simulink subsystem "induction_motor_model"  (R2024b)
settings: Solver=VariableStepAuto  StartTime=0.0  StopTime=10.0  RelTol=1e-3
model mask{A=400, f=50}
  mask prompts: A "Amplitude (V)"; f "Frequency (Hz)"
settings Model: Creator=antoinedaniel  LastModifiedBy=antoinedaniel

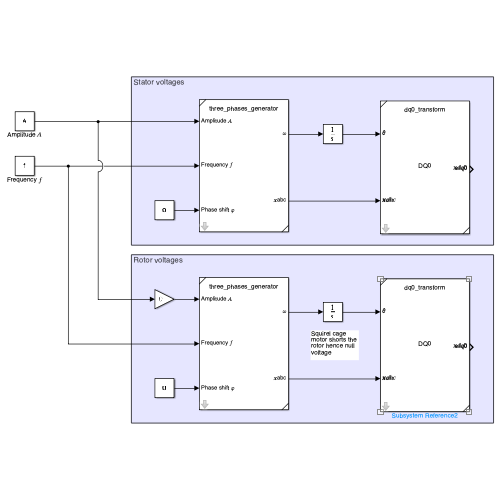
[thumbnail: Simulink's stored preview of the top-level diagram]
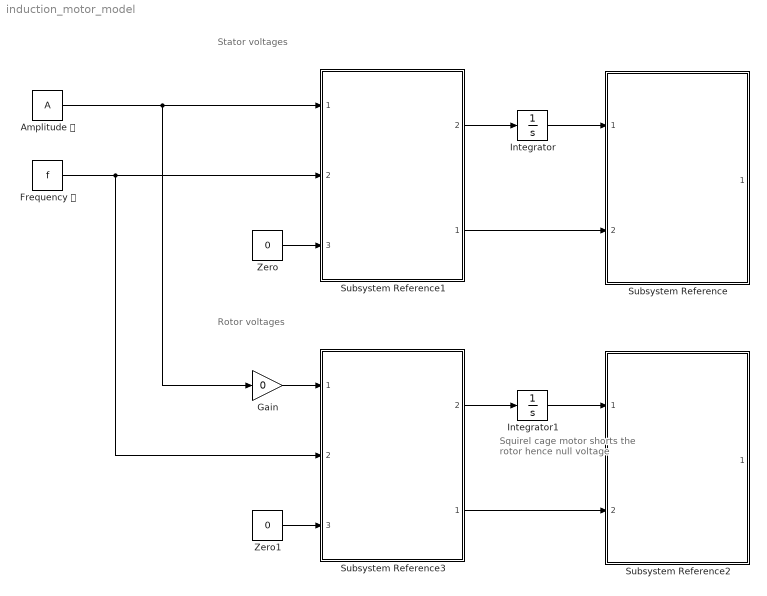
== system induction_motor_model ==
  note: Stator voltages
  note: Squirel cage motor shorts the rotor hence null voltage
  note: Rotor voltages
  Amplitude 𝐴 : Constant  Value=A
  Frequency 𝑓 : Constant  Value=f
  Gain : Gain  Gain=0
  Integrator : Integrator
  Integrator1 : Integrator
  Subsystem Reference : Subsystem  ReferencedSubsystem=dq0_transform  SignConv=Negative
  Subsystem Reference1 : Subsystem  ReferencedSubsystem=three_phases_generator
      settings: PortSchema="{\"entries\":[{\"content\":{\"sides\":[{\"content\":{\"connectorIds\":[\"In1\",\"In2\",\"In3\"]},\"type\":\"ConnectorPlacement.EquallySpacedRectSide\",\"uuid\":\"83e992db-efbf-4d18-ab7d-fa4d5e1c88d1\"},{\"content\":{\"connectorIds\":[\"Out2\",\"Out1\"],\"side\":\"RIGHT\"},\"type\":\"ConnectorPlacement.EquallySpacedRectSide\",\"uuid\":\"656c653f-2ce0-4e40-9b0c-6992e4a2161f\"},{\"content\":{\"side\":\"TOP\"},\"type\":\"ConnectorPlacement.EquallySpacedRectSide\",\"uuid\":\"72561826-dcd0-46fd-8f68-d4b433a3570d\"}]},\"type\":\"ConnectorPlacement.EquallySpacedConnector\",\"uuid\":\"af8caae1-e993-43bd-9cc3-dee22ee1edeb\"}],\"packageUris\":[\"http://schema.mathworks.com/mf0/Connector/R2020b\"],\"version\":\"1.0\"}"
  Subsystem Reference2 : Subsystem  ReferencedSubsystem=dq0_transform  SignConv=Negative
  Subsystem Reference3 : Subsystem  ReferencedSubsystem=three_phases_generator
      settings: PortSchema="{\"entries\":[{\"content\":{\"sides\":[{\"content\":{\"connectorIds\":[\"In1\",\"In2\",\"In3\"]},\"type\":\"ConnectorPlacement.EquallySpacedRectSide\",\"uuid\":\"83e992db-efbf-4d18-ab7d-fa4d5e1c88d1\"},{\"content\":{\"connectorIds\":[\"Out2\",\"Out1\"],\"side\":\"RIGHT\"},\"type\":\"ConnectorPlacement.EquallySpacedRectSide\",\"uuid\":\"656c653f-2ce0-4e40-9b0c-6992e4a2161f\"},{\"content\":{\"side\":\"TOP\"},\"type\":\"ConnectorPlacement.EquallySpacedRectSide\",\"uuid\":\"72561826-dcd0-46fd-8f68-d4b433a3570d\"}]},\"type\":\"ConnectorPlacement.EquallySpacedConnector\",\"uuid\":\"af8caae1-e993-43bd-9cc3-dee22ee1edeb\"}],\"packageUris\":[\"http://schema.mathworks.com/mf0/Connector/R2020b\"],\"version\":\"1.0\"}"
  Zero : Constant  Value=0  OutDataTypeStr=Inherit: Inherit via back propagation
  Zero1 : Constant  Value=0  OutDataTypeStr=Inherit: Inherit via back propagation
  wires:
  Zero/1 -> Subsystem Reference1/3
  Subsystem Reference1/1 -> Subsystem Reference/2
  Subsystem Reference1/2 -> Integrator/1
  Integrator/1 -> Subsystem Reference/1
  Amplitude 𝐴/1 -> Gain/1, Subsystem Reference1/1
  Frequency 𝑓/1 -> Subsystem Reference3/2, Subsystem Reference1/2
  Subsystem Reference3/2 -> Integrator1/1
  Zero1/1 -> Subsystem Reference3/3
  Subsystem Reference3/1 -> Subsystem Reference2/2
  Integrator1/1 -> Subsystem Reference2/1
  Gain/1 -> Subsystem Reference3/1
